simulink model "gravity"  (Simulink 7.7)
settings: Solver=FixedStepDiscrete  StartTime=0.0  StopTime=inf  FixedStep=0.25  RelTol=1e-3
undefined symbols (not defined in the file): darwinop_communication_setup
libraries: simulink x4, lib_darwinop x1
settings Model: Creator=florent  LastModifiedBy=eleve
settings DataIOCC: SignalLoggingSaveFormat=Dataset
settings OptimizationCC: ExpressionDepthLimit=128  OptimizeModelRefInitCode=on  LifeSpan=Inf
settings DebuggingCC: FcnCallInpInsideContextMsg=Enable All
settings HardwareCC: ProdEndianess=LittleEndian  ProdHWDeviceType=Generic->32-bit Embedded Processor
settings RTWCC: SystemTargetFile=darwinoplib.tlc  TemplateMakefile=darwinoplib.tmf  Description=DarwinOP code generator  ProcessScript=darwinoplib_make_rtw_hook  TargetLang=C++
settings CodeAppCC: IgnoreCustomStorageClasses=off  CustomSymbolStrType=$N$R$M_T
settings STFCustomTargetCC: CombineOutputUpdateFcns=on  ERTCustomFileBanners=on  SupportContinuousTime=off  SupportNonInlinedSFcns=off  SystemTargetFile=darwinoplib.tlc
settings ERTTargetCC: MultiwordLength=2048  ParMdlRefBuildCompliant=off  CompOptLevelCompliant=off  ERTFirstTimeCompliant=off  ModelStepFunctionPrototypeControlCompliant=off  CPPClassGenCompliant=off  InlinedParameterPlacement=NonHierarchical  ERTCustomFileTemplate=darwinoplib_main.tlc  ConvertIfToSwitch=off  SuppressUnreachableDefaultCases=off
settings CustomProperty: DataType=string  Value=192.168.123.1

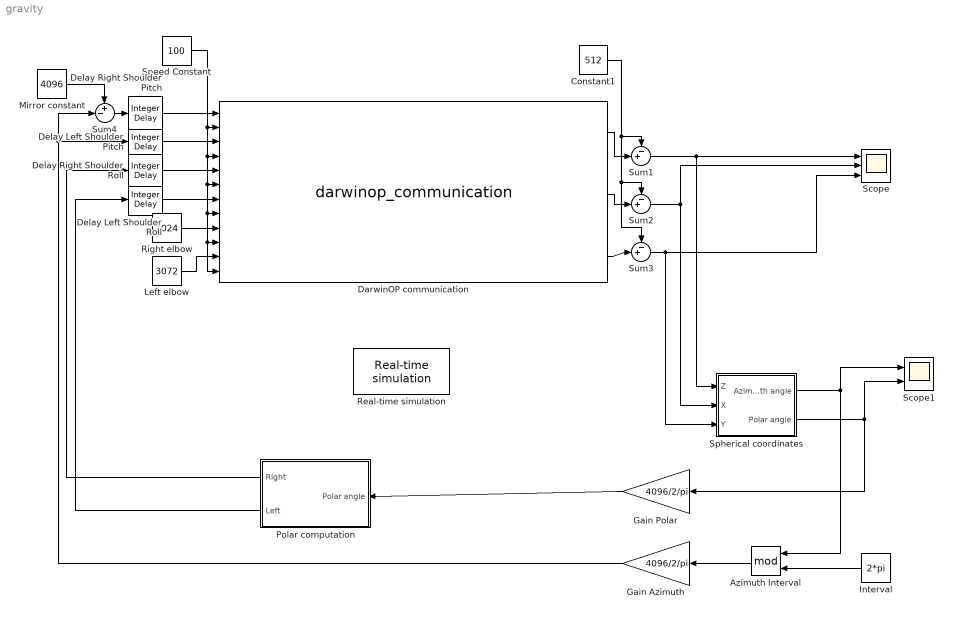
== system gravity ==
  Azimuth Interval : Math  Operator=mod  SaturateOnIntegerOverflow=on
  Constant1 : Constant  Value=512
  DarwinOP communication : M-S-Function  StartFcn=darwinop_communication_setup('StartFcn');  StopFcn=darwinop_communication_setup('StopFcn');  FunctionName=darwinop_communication  Parameters=IP,Port,Protocol,Timeout,Frame,ReadIndex,WriteIndex  mask{IP=192.168.123.1, Port=1234, Protocol=tcp, Timeout=0.25, Frame=[ 3 1 30 4 0 0 0 0 3 2 30 4 0 0 0 0 3 3 30 4 0 0 0 0 3 4 30 4 0 0 0 0 3 5 30 4 0 0 0 0 3 6 30 4 0 0 0 0 2 200 44 6], ReadIndex=[ 1 2;3 2;5 2], WriteIndex=[ 5 2;7 2;13 2;15 2;21 2;23 2;29 2;31 2;37 2;39 2;45 2;47 2]}
      settings: DeleteFcn=darwinop_communication_setup('DeleteFcn');  ModelCloseFcn=darwinop_communication_setup('ModelCloseFcn');  NameChangeFcn=darwinop_communication_setup('NameChangeFcn');  OpenFcn=darwinop_communication_setup('OpenFcn');
      mask StyleString: edit,edit,popup(tcp|udp),edit,edit,edit,edit
      mask Display:
      | image(imread('darwin-blk.jpg'))
      | 
      | port_label('output',1,'Sub controller(200)/ACC X')
      | port_label('output',2,'Sub controller(200)/ACC Y')
      | port_label('output',3,'Sub controller(200)/ACC Z')
      | 
      | port_label('input',1,'Right Shoulder Pitch(1)/Goal Position')
      | port_label('input',2,'Right Shoulder Pitch(1)/Moving Speed')
      | port_label('input',3,'Left Shoulder Pitch(2)/Goal Position')
      | port_label('input',4,'Left Shoulder Pitch(2)/Moving Speed')
      | port_label('input',5,'Right Shoulder Roll(3)/Goal Position')
      | port_label('input',6,'Right Shoulder Roll(3)/Moving Speed')
      | port_label('input',7,'Left Shoulder Roll(4)/Goal Position')
      | port_label('input',8,'Left Shoulder Roll(4)/Moving Speed')
      | port_label('input',9,'Right Elbow(5)/Goal Position')
      | port_label('input',10,'Right Elbow(5)/Moving Speed')
      | port_label('input',11,'Left Elbow(6)/Goal Position')
      | port_label('input',12,'Left Elbow(6)/Moving Speed')
  Delay Left Shoulder Pitch : simulink/Discrete/Integer Delay  NumDelays=1  vinit=2048  samptime=-1
  Delay Left Shoulder Roll : simulink/Discrete/Integer Delay  NumDelays=1  vinit=2048  samptime=-1
  Delay Right Shoulder Pitch : simulink/Discrete/Integer Delay  NumDelays=1  vinit=2048  samptime=-1
  Delay Right Shoulder Roll : simulink/Discrete/Integer Delay  NumDelays=1  vinit=2048  samptime=-1
  Gain Azimuth : Gain  Gain=4096/2/pi
  Gain Polar : Gain  Gain=4096/2/pi
  Interval : Constant  Value=2*pi
  Left elbow : Constant  Value=3072
  Mirror constant : Constant  Value=4096
  Polar computation : Subsystem
  Real-time simulation : lib_darwinop/Real-time simulation  TimeScalingFactor=1
  Right elbow : Constant  Value=1024
  Scope : Scope  NumInputPorts=3
      settings: YMin=1000~-100~-700  YMax=3000~475~200
  Scope1 : Scope  NumInputPorts=2
      settings: YMin=-3.141592653589793~-3.141592653589793  YMax=3.141592653589793~3.141592653589793
  Speed Constant : Constant  Value=100
  Spherical coordinates : Subsystem
  Sum1 : Sum  Inputs=-+|
  Sum2 : Sum  Inputs=-+|
  Sum3 : Sum  Inputs=-+|
  Sum4 : Sum  Inputs=+-|
  wires:
  DarwinOP communication/1 -> Sum1/2
  Sum1/1 -> Scope/1, Spherical coordinates/1(Z)
  DarwinOP communication/2 -> Sum2/2
  Sum2/1 -> Scope/2, Spherical coordinates/2(X)
  DarwinOP communication/3 -> Sum3/2
  Sum3/1 -> Spherical coordinates/3(Y), Scope/3
  Constant1/1 -> Sum1/1, Sum2/1, Sum3/1
  Mirror constant/1 -> Sum4/1
  Gain Azimuth/1 -> Delay Left Shoulder Pitch/1, Sum4/2
  Speed Constant/1 -> DarwinOP communication/2, DarwinOP communication/4, DarwinOP communication/6, DarwinOP communication/8, DarwinOP communication/10, DarwinOP communication/12
  Azimuth Interval/1 -> Gain Azimuth/1
  Interval/1 -> Azimuth Interval/2
  Sum4/1 -> Delay Right Shoulder Pitch/1
  Right elbow/1 -> DarwinOP communication/9
  Left elbow/1 -> DarwinOP communication/11
  Spherical coordinates/1(Azimuth angle) -> Scope1/1, Azimuth Interval/1
  Spherical coordinates/2(Polar angle) -> Scope1/2, Gain Polar/1
  Gain Polar/1 -> Polar computation/1(Polar angle)
  Polar computation/1(Right) -> Delay Right Shoulder Roll/1
  Polar computation/2(Left) -> Delay Left Shoulder Roll/1
  Delay Right Shoulder Pitch/1 -> DarwinOP communication/1
  Delay Left Shoulder Pitch/1 -> DarwinOP communication/3
  Delay Left Shoulder Roll/1 -> DarwinOP communication/7
  Delay Right Shoulder Roll/1 -> DarwinOP communication/5

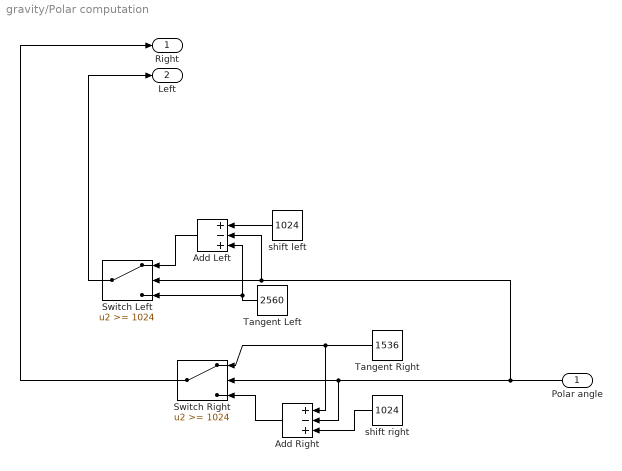
== system gravity/Polar computation ==
  Polar angle : Inport
  Add Left : Sum  Inputs=+-+
  Add Right : Sum  Inputs=+-+
  Switch Left : Switch  Threshold=1024
  Switch Right : Switch  Threshold=1024
  Tangent Left : Constant  Value=2560
  Tangent Right : Constant  Value=1536
  shift left : Constant  Value=1024
  shift right : Constant  Value=1024
  Right : Outport
  Left : Outport  Port=2
  wires:
  Add Left/1 -> Switch Left/1
  Switch Right/1 -> Right/1
  Switch Left/1 -> Left/1
  shift left/1 -> Add Left/1
  Tangent Right/1 -> Add Right/1, Switch Right/1
  Polar angle/1 -> Add Left/2, Switch Left/2, Add Right/2, Switch Right/2
  shift right/1 -> Add Right/3
  Add Right/1 -> Switch Right/3
  Tangent Left/1 -> Add Left/3, Switch Left/3

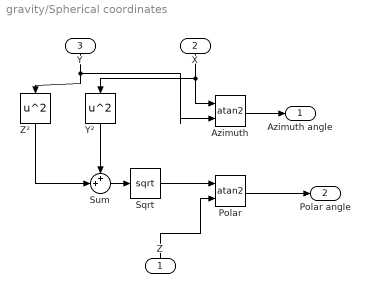
== system gravity/Spherical coordinates ==
  Z : Inport
  X : Inport  Port=2
  Y : Inport  Port=3
  Azimuth : Trigonometry  Operator=atan2
  Polar : Trigonometry  Operator=atan2
  Sqrt : Sqrt  SaturateOnIntegerOverflow=on
  Sum : Sum  Inputs=++|
  Y² : Math  Operator=square  SaturateOnIntegerOverflow=on
  Z² : Math  Operator=square  SaturateOnIntegerOverflow=on
  Azimuth angle : Outport
  Polar angle : Outport  Port=2
  wires:
  Y/1 -> Azimuth/2, Z²/1
  X/1 -> Y²/1, Azimuth/1
  Z/1 -> Polar/2
  Sqrt/1 -> Polar/1
  Sum/1 -> Sqrt/1
  Z²/1 -> Sum/2
  Y²/1 -> Sum/1
  Polar/1 -> Polar angle/1
  Azimuth/1 -> Azimuth angle/1
